simulink library "rtlsdr_book_library"  (R2018a)
settings: Solver=ode45  StartTime=0.0  StopTime=10.0  RelTol=1e-3  EnableMultiTasking=on
undefined symbols (not defined in the file): costas, den, dfilt, fdesignblkfcn, frm, gcbh, iir, num, rtlsdr_frmsize, rtlsdr_fs, src
libraries: dspsigops x6, commsynccomp2 x4, dspsrcs4 x2, dspstat3 x2, dspobslib x2, simulink_extras x2, dspmtrx3 x2, dsparch4 x1, $bdroot x1, dspspect3 x1, commrflib2 x1
(part 5 of 5)

== system rtlsdr_book_library/Sync Tools for Analogue Comms/Phase Locked Loop Demodulator/Reduce Output Rate/Enabled Subsystem ==
  In1 : Inport
  Enable : EnablePort
  Out1 : Outport
  wires:
  In1/1 -> Out1/1

== matlab function rtlsdr_book_library/Data Comms Sources and Sinks/Image Transfer Binary Source/MATLAB Function ==
  data: count_lim input; master_frame input; frame_output output
function frame_output = fcn(count_lim, master_frame)
persistent column_count;

if isempty(column_count)
    column_count = 1;
end
frame_output = master_frame(:,column_count);
column_count = column_count +1;
if column_count == count_lim+1
    column_count = 1;
end

% %frame_output = [1,1:length(master_frame)-1];
end

== matlab function rtlsdr_book_library/Data Comms Sources and Sinks/Image Reconstruction/Image Reconstruction ==
  data: frame_in input; binary_len input
%% Image Transfer: Image Reconstruction
% This function is used to process received frames of data and rebuild the
% image that has been transferred. Once the appropriate number of frames
% has been retrieved, the image is then plotted in a figure for the user to
% observe.

function message_decoder_img_transfer(frame_in, binary_len)

%% FUNCTION SETUP
% functions that cannot be compiled
coder.extrinsic('assignin')
coder.extrinsic('get_param')
coder.extrinsic('set_param')
coder.extrinsic('num2str')
coder.extrinsic('bdroot')
coder.extrinsic('gcs')
coder.extrinsic('disp')

%% PROTOCOL PARAMETERS
% make frame length persistent across function calls
persistent frame_len;
% initialise variable on first call to function
if isempty(frame_len)
    frame_len = 1000;                                                      % total length of a frame
end

%% IMAGE RECONSTRUCTION PARAMETERS
% make variables persistent across function calls
persistent image seq_num_storage valid_seq_num prev_seqnum sequence_num...
    initial_op_flag seqnum_lock seqnum_countenable;

% initialise variables
img_rx = 0;                                                                % variable that will hold each input frame
data_len = 0;                                                              % variable to store data length of each frame
header_len = 0;                                                            % variable to store header length of each frame
img_pixels_x = 100;                                                        % default value for image width
img_pixels_y = 100;                                                        % default value for image height

% initialise persistent variables on first call to function
if isempty(initial_op_flag)
    initial_op_flag = 0;                                                   % initialise output flag for information message to print
end
if isempty(image)
    image = zeros(img_pixels_x,img_pixels_y);                              % initialise image storage variable
    image(1:img_pixels_x,1:img_pixels_y) = uint8(255);                     % set matrix values to 255 - making default matrix a white background
end
if isempty(seq_num_storage)
    seq_num_storage = zeros(1,img_pixels_x);                               % initialise sequence number storage
end
if isempty(valid_seq_num)
    valid_seq_num = 1;                                                     % set valid sequence number flag high
end
if isempty(prev_seqnum)
    prev_seqnum = zeros(1,4);                                              % initialise previous sequence number vector for storage of past values
end
if isempty(sequence_num)
    sequence_num = 1;                                                      % initialise sequence number to store individual frame's sequence number
end
if isempty(seqnum_lock)
    seqnum_lock = 0;                                                       % set sequence number lock low
end
if isempty(seqnum_countenable)
    seqnum_countenable = 0;                                                % set sequence number count enable low
end

% assert specific variables for code generation
assert (data_len <= frame_len);
assert (header_len <= frame_len);
assert (img_rx <= frame_len);

% provide bounds for size of variables 'payload' and 'pixel_column'
coder.varsize ('payload', 1000);
coder.varsize ('pixel_column', [1 100]);

%% HEADER PARAMETERS
persistent seq_num_bit_len end_flag_bit_len header_bit_len payload_bit_len pad_bit_len;
if isempty(seq_num_bit_len)
    seq_num_bit_len = 8;                                                   % # of bits in header - frame sequence number length
end
if isempty(end_flag_bit_len)
    end_flag_bit_len = 1;                                                  % # of bits in header - end packet flag length
end
if isempty(header_bit_len)
    header_bit_len = 8;                                                    % # of bits in header - header length
end
if isempty(payload_bit_len)
    payload_bit_len = 10;                                                  % # of bits in header - payload length
end
if isempty(pad_bit_len)
    pad_bit_len = 9;                                                       % # of bits in header - padding length
end

%% Frame Header Structure
%-------------------------------------------------------------------------%
% Frame Header- [Preamble, sequence number, end flag, header length,
%                payload length, padding length]
%-------------------------------------------------------------------------%

% set the preamble in unipolar form - used at the beginning of each frame
preamble = [1,1,1,1,1,1,1,1,1,1,1,1,1,1,1,0,0,0,0,0,0,1,1,1,1,1,1,0,0,0,1,1,1,0,0,0,1,1,1];
preamble_len = length(preamble);                                           % calculate decimal length of the preamble sequence
preamble_pad_len = rem(preamble_len,2);                                    % determine length of preamble padding

% determine the starting index positions for the fields of the header
seq_num_pos = preamble_len + preamble_pad_len+1;                           % sequence number starts after the preamble
end_flag_pos = seq_num_pos + seq_num_bit_len;                              % end flag (indicating last frame) starts after the sequence number
header_len_pos = end_flag_pos + end_flag_bit_len;                          % header length starts after the end flag
payload_len_pos = header_len_pos + header_bit_len;                         % payload length starts after the header length
pad_len_pos = payload_len_pos + payload_bit_len;                           % padding length starts after the payload length

% typecast the input frame to uint8 and store in 'img_rx'
img_rx = uint8(frame_in);

%-------------------------------------------------------------------------%
% Store and use previous sequence numbers to obtain a sequence lock signal

% prev_seqnum stores the current and last three sequence numbers
for i = 4:-1:2
    prev_seqnum(i) = prev_seqnum(i-1);                                     % shift previous sequence numbers in register - oldest shifted out
end
prev_seqnum(1) = sequence_num;                                             % store current sequence number before next current value is obtained

if (prev_seqnum(4)+1==prev_seqnum(3) && ...                                % if all 4 values are an increment of each other in the correct order
        prev_seqnum(3)+1==prev_seqnum(2) && ...
        prev_seqnum(2)+1==prev_seqnum(1) )
    
    seqnum_lock = prev_seqnum(1);                                          % set the lock to the current sequence number
    seqnum_countenable = 1;                                                % set the count enable to allow the lock signal to increment
end
if seqnum_countenable == 1                                                 % if lock enable signal is high
    seqnum_lock = seqnum_lock+1;                                           % increment the lock signal
end

%-------------------------------------------------------------------------%
% Extract and convert the header fields to decimal values

% obtain the sequence number stored in the current frame
sequence_num = bi2de(double(img_rx(seq_num_pos:seq_num_pos+seq_num_bit_len-1)'),'left-msb');

% obtain the header length — used to determine payload location
header_len = bi2de(double(img_rx(header_len_pos:header_len_pos+header_bit_len-1)'),'left-msb');

if header_len ~= 76                                                        % if header length has been recovered with errors, set to a default value
    header_len = 76;
end

% obtain the payload length — used to recover the image data in the frame
payload_len = bi2de(double(img_rx(payload_len_pos:payload_len_pos+payload_bit_len-1)'),'left-msb');

if payload_len ~= 924                                                      % if payload length has been recovered with errors, set to a default value
    payload_len = 924;
end

% obtain the padding length — used to calculate data length
padding_len = bi2de(double(img_rx(pad_len_pos:pad_len_pos+pad_bit_len-1)'),'left-msb');

% calculate data length from other header fields
data_len = payload_len - padding_len;

if data_len ~= 800                                                         % if data length has been recovered with errors, set to a default value
    data_len = 800;
end
%-------------------------------------------------------------------------%
% Find data positions and extract data from current frame

data_start = header_len+1;                                                 % find data start
data_end = header_len+data_len;                                            % find data end
data = img_rx(data_start:data_end);                                        % extract data from frame

%-------------------------------------------------------------------------%
% Search for the first valid frame

% display the information message before a frame is found
if initial_op_flag == 0
    disp('Searching for first frame...');
    initial_op_flag = 1;
end

% if sequence number is out of normal bounds
if sequence_num < 1 || sequence_num > 100                                  % sequence numbers should be between 1 & 100 for 100 column images
    if seqnum_countenable == 1                                             % if count enable for lock is high
        sequence_num = seqnum_lock;                                        % allow sequence number to be obtained from sequence number lock
    else
        valid_seq_num  = 0;                                                % if the count enable is low and hence not locked, don't recover the frame
    end
end

%-------------------------------------------------------------------------%
% If the conditions are met, extract pixel data to decimal image column

pixel_column = zeros(1,img_pixels_y);                                      % declare variable for data storage

if valid_seq_num == 1 && seqnum_lock < 100                                 % if the recovered sequence number is value and sequence number lock is less than end of frame
    disp([' Picture Column Number: ',num2str(sequence_num)]);              % indicate in command window which column has just been received using current sequence number
    
    % recover each pixel of the column from the data
    for count = 1:1:img_pixels_y
        pixel_binary = data((((count-1)*binary_len)+1):binary_len*count);  % use 'count' to extract one byte per pixel
        pixel_column(count) = bi2de(double(pixel_binary'),'left-msb');             % store decimal value of pixel in column
    end
    
    % check if the current frame (column) has been received before or not
    if seq_num_storage(sequence_num) == 0
        seq_num_storage(sequence_num) = sequence_num;                      % if not, record sequence number
        image(:,sequence_num) = pixel_column;                              % save received column of pixels into image variable using current sequence number
    end
end
if valid_seq_num == 0
    valid_seq_num = 1;                                                     % reset valid_seq_num if it has been set low
end

% if 100 frames have been received and processed
if seqnum_lock >= 100
    assignin('base', 'image', image);                                      % save image to MATLAB workspace
    set_param(bdroot, 'SimulationCommand', 'pause')                        % pause simulation to run plotting callback
    
    % *callback runs, then model execution continued*
    
    % reset persistent variables
    seq_num_storage = zeros(1,100);
    %image = zeros(100,100);
    image(1:100,1:100) = uint8(255);
    seqnum_lock = 0;
    seqnum_countenable = 0;
    prev_seqnum = zeros(1,4);
end
%-------------------------------------------------------------------------%
end

== matlab function rtlsdr_book_library/Sync Tools for Digital Comms/Coarse Freq Correction/Find Frequency Offset ==
  data: Frame_width input; freq_offset output; Frame_period input; Peak_index input; Signal_width input
%% Frequency offset calculation
% The code in this function takes the inputs, and uses them to calculate 
% the frequency offset required to synchronise the input signal to baseband. 
%-------------------------------------------------------------------------%
function freq_offset = fcn(Frame_width,Frame_period,Peak_index,Signal_width)
% Logic to compute required index offset value
if Peak_index > Signal_width/2
    offset = (Signal_width+1)-Peak_index;
else
    offset = 1-Peak_index;
end

% Convert offset to a frequency shift value.
% calculate sample time
Ts = Frame_period(1)/Frame_width;
% calculate frequency resolution of the FFT signal
freq_resolution = 1/(Ts*Signal_width);
% compute frequency offset using this value
freq_offset = offset * freq_resolution/4;

== matlab function rtlsdr_book_library/Data Comms Sources and Sinks/ASCII Decoding/Binary to ASCII ==
  data: msg input; msg_len input; ascii_len input
function msg_decoder(msg,msg_len,ascii_len)

% assert limits of msg_len for compiler
assert(msg_len>=1)
assert(msg_len<=2000)

% enable functions to be used by compiler
coder.extrinsic('uicontrol')
coder.extrinsic('disp')
coder.extrinsic('num2str')

% initialise output word with zeros
word = char(zeros(1,msg_len));

% convert ascii bits to ascii chars, save to string
for count = 1:1:msg_len
    char_bin = msg((((count-1)*ascii_len)+1):ascii_len*count)';
    word(count) = char(bi2de(double(char_bin),'left-msb'));
end
disp(word);    
end

== matlab function rtlsdr_book_library/Data Comms Sources and Sinks/  ASCII Transfer Binary Source/MATLAB Function ==
  data: count_lim input; master_frame input; frame_output output
function frame_output = fcn(count_lim, master_frame)
persistent column_count;                        % set variable to persist across function calls

if isempty(column_count)                        % check if the column_count variable has been initialised
    column_count = 1;                           % initialise if it hasn't been already
end

frame_output = master_frame(:,column_count);    % output each frame individually
column_count = column_count +1;                 % increment the count for the next function call

if column_count == count_lim+1                  % check if the max # of frames has been reached
    column_count = 1;                           % reset the counter to repeat the process
end
end
